simulink model "ACCfinall"  (Simulink 8.4)
settings: Solver=ode45  StartTime=0.0  StopTime=200.0  RelTol=1e-3
undefined symbols (not defined in the file or in its folder): sigbuilder_block
libraries: simulink x1
settings Model: Creator=asim  LastModifiedBy=asim
settings DataIOCC: SignalLoggingSaveFormat=Dataset
settings OptimizationCC: ExpressionDepthLimit=128
settings DebuggingCC: UnderspecifiedInitializationDetection=Simplified  MergeDetectMultiDrivingBlocksExec=error  SolverPrmCheckMsg=none  FcnCallInpInsideContextMsg=EnableAllAsError  StateNameClashWarn=none
settings GRTTargetCC: CombineOutputUpdateFcns=on  GRTInterface=off

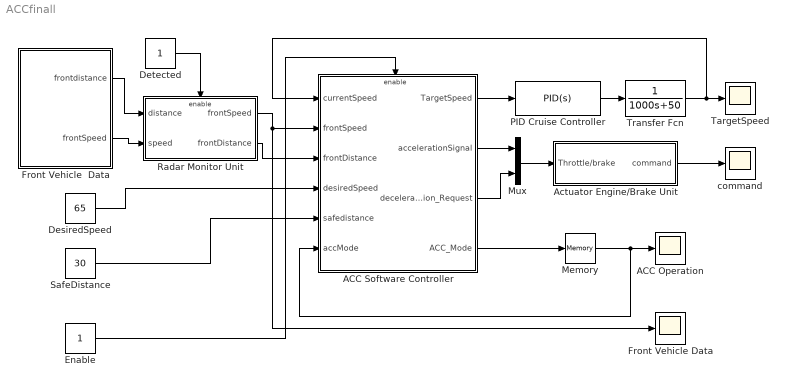
== system ACCfinall ==
  ACC Operation : Scope
      settings: TimeRange=10  YMin=0  YMax=3  SaveName=ScopeData3
  "ACC Software Controller " : Subsystem
  Actuator Engine/Brake Unit : Subsystem
  DesiredSpeed : Constant  Value=65
  "Detected " : Constant
  Enable : Constant
  Front Vehicle  Data : Subsystem  Tag=STV Subsys  LoadFcn=sigbuilder_block('load');  StartFcn=sigbuilder_block('start');  StopFcn=sigbuilder_block('stop');  ClipboardFcn=sigbuilder_block('clipboard');  mask(Sigbuilder block){}
      mask help: Simulink:masks:SigbuilderBlock_MD
      mask init:
      | if ~strcmp(get_param(bdroot(gcbh),'SimulationStatus'),'stopped') tuvar = sigbuilder_block('maskInit'); end
      settings: CopyFcn=sigbuilder_block('copy');  DeleteFcn=sigbuilder_block('delete');  ModelCloseFcn=sigbuilder_block('modelClose');  PreSaveFcn=sigbuilder_block('preSave');  PauseFcn=sigbuilder_block('pause');  ContinueFcn=sigbuilder_block('continue');  NameChangeFcn=sigbuilder_block('namechange');  OpenFcn=sigbuilder_block('open',[410.25 112.5 550.5 394.5 ]);  CloseFcn=sigbuilder_block('close');
      mask Display: plot(0, 0, 100, 100,[2, 2, 32, 32, 2], [68, 8, 8, 68, 68],[32, 2], [38, 38], [32, 19, 2],[53, 60, 44], [32, 17, 17, 2],[16, 16, 31, 31]);txt = getActiveGroup(gcbh);text(2, 100, txt,'verticalAlignment', 'top');
  Front Vehicle Data : Scope
  Memory : Memory  InheritSampleTime=on
  Mux : Mux  Inputs=2
  PID Cruise Controller : simulink/Continuous/PID Controller  Controller=PID  TimeDomain=Continuous-time  SampleTime=-1  IntegratorMethod=Forward Euler  FilterMethod=Forward Euler  Form=Parallel  P=65.9263869879216  I=5.57652865052723  D=-273.538535319166  N=0.241013160763614  InitialConditionSource=internal  InitialConditionForIntegrator=0  InitialConditionForFilter=0  ExternalReset=none  LimitOutput=off  UpperSaturationLimit=inf  LowerSaturationLimit=-inf  LinearizeAsGain=on  AntiWindupMode=none  Kb=1  TrackingMode=off  Kt=1  PParamMin=[]  PParamMax=[]  IParamMin=[]  IParamMax=[]  DParamMin=[]  DParamMax=[]  NParamMin=[]  NParamMax=[]  KbParamMin=[]  KbParamMax=[]  KtParamMin=[]  KtParamMax=[]  POutMin=[]  POutMax=[]  IOutMin=[]  IOutMax=[]  DOutMin=[]  DOutMax=[]  NOutMin=[]  NOutMax=[]  KbOutMin=[]  KbOutMax=[]  KtOutMin=[]  KtOutMax=[]  IntegratorOutMin=[]  IntegratorOutMax=[]  FilterOutMin=[]  FilterOutMax=[]  SumOutMin=[]  SumOutMax=[]  SumI1OutMin=[]  SumI1OutMax=[]  SumI2OutMin=[]  SumI2OutMax=[]  SumI3OutMin=[]  SumI3OutMax=[]  SumDOutMin=[]  SumDOutMax=[]  SaturationOutMin=[]  SaturationOutMax=[]  IntegratorContinuousStateAttributes=''  IntegratorStateMustResolveToSignalObject=off  IntegratorRTWStateStorageClass=Auto  FilterContinuousStateAttributes=''  FilterStateMustResolveToSignalObject=off  FilterRTWStateStorageClass=Auto  DifferentiatorICPrevScaledInput=0  DifferentiatorOutMin=[]  DifferentiatorOutMax=[]  UseFilter=on
  Radar Monitor Unit : Subsystem
  SafeDistance : Constant  Value=30
  TargetSpeed : Scope
      settings: YMin=0  YMax=70
  Transfer Fcn : TransferFcn  Denominator=[1000 50]
  command : Scope
      settings: SaveName=ScopeData2
  wires:
  "ACC Software Controller "/1(TargetSpeed) -> PID Cruise Controller/1
  Transfer Fcn/1 -> TargetSpeed/1, "ACC Software Controller "/1(currentSpeed)
  Radar Monitor Unit/2(frontDistance) -> "ACC Software Controller "/3(frontDistance)
  PID Cruise Controller/1 -> Transfer Fcn/1
  "ACC Software Controller "/4(ACC_Mode) -> Memory/1
  Memory/1 -> ACC Operation/1, "ACC Software Controller "/6(accMode)
  "ACC Software Controller "/2(accelerationSignal) -> Mux/1
  "ACC Software Controller "/3(deceleration_Request) -> Mux/2
  Mux/1 -> Actuator Engine/Brake Unit/1(Throttle/brake)
  Actuator Engine/Brake Unit/1(command) -> command/1
  Front Vehicle  Data/1(frontdistance) -> Radar Monitor Unit/1(distance)
  Radar Monitor Unit/1(frontSpeed) -> "ACC Software Controller "/2(frontSpeed), Front Vehicle Data/1
  DesiredSpeed/1 -> "ACC Software Controller "/4(desiredSpeed)
  SafeDistance/1 -> "ACC Software Controller "/5(safedistance)
  Enable/1 -> "ACC Software Controller "/Enable
  "Detected "/1 -> Radar Monitor Unit/Enable
  Front Vehicle  Data/2(frontSpeed) -> Radar Monitor Unit/2(speed)

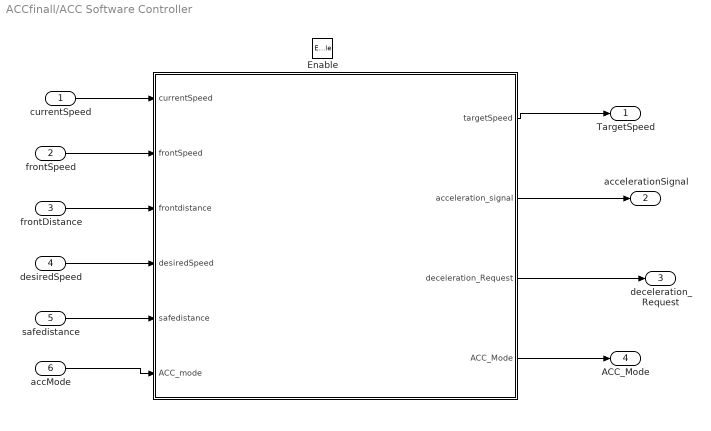
== system ACCfinall/ACC Software Controller  ==
  currentSpeed : Inport
  frontSpeed : Inport  Port=2
  frontDistance : Inport  Port=3
  desiredSpeed : Inport  Port=4
  safedistance : Inport  Port=5
  accMode : Inport  Port=6
  Enable : EnablePort
  "          " : MATLAB Function  TreatAsAtomicUnit=on
  TargetSpeed : Outport
  accelerationSignal : Outport  Port=2
  deceleration_Request : Outport  Port=3
  ACC_Mode : Outport  Port=4
  wires:
  "          "/1(targetSpeed) -> TargetSpeed/1
  currentSpeed/1 -> "          "/1(currentSpeed)
  "          "/2(acceleration_signal) -> accelerationSignal/1
  "          "/4(ACC_Mode) -> ACC_Mode/1
  "          "/3(deceleration_Request) -> deceleration_Request/1
  frontSpeed/1 -> "          "/2(frontSpeed)
  frontDistance/1 -> "          "/3(frontdistance)
  desiredSpeed/1 -> "          "/4(desiredSpeed)
  safedistance/1 -> "          "/5(safedistance)
  accMode/1 -> "          "/6(ACC_mode)

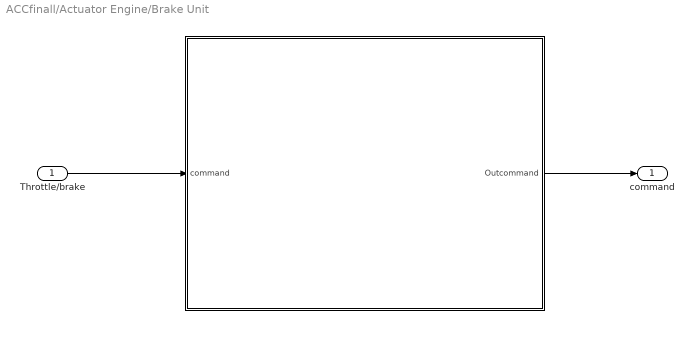
== system ACCfinall/Actuator Engine/Brake Unit ==
  Throttle/brake : Inport
  "          " : MATLAB Function  TreatAsAtomicUnit=on
  command : Outport
  wires:
  "          "/1(Outcommand) -> command/1
  Throttle/brake/1 -> "          "/1(command)

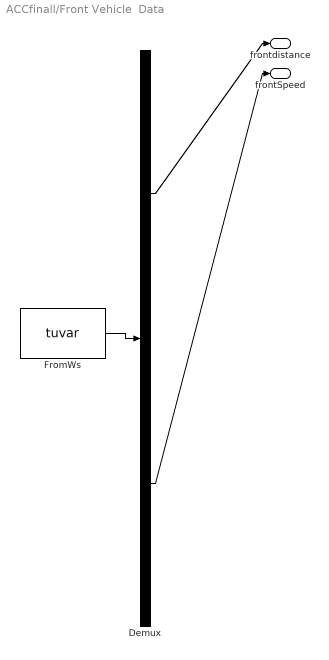
== system ACCfinall/Front Vehicle  Data ==
  Demux : Demux  Tag=STV Demux  Outputs=2
  FromWs : FromWorkspace  Tag=STV FromWs  VariableName=tuvar  SampleTime=0  SigBuilderData=DataTag0  VnvData=DataTag1
      SigBuilderData=|
      | common.afterFinalStr = 'Extrapolate'
      | common.sampleTime = 0
      | dataSet.timeRange = [10 100]
      | dataSet.name = 'Front Vehicle '
      | sbobj.Groups.Name = 'Front Vehicle '
      | sbobj.Groups.Signals(1).Name = 'frontdistance'
      | sbobj.Groups.Signals(1).XData = [10 11 11 12 12 13 13 14 14 15 15 16 16 17 17 18 18 19 19 20 20 21 21 22 22 23 23 24 24 25 25 26 26 27 27 28 28 29 29 30 30 31 31 32 32 33 33 34 34 35 35 36 36 37 37 38 38 39 39 40 40 41 41 42 42 43 43 44 44 45 45 46 46 47 47 48 48 49 49 50 50 51 51 52 52 53 53 54 54 55 55 56 56 57 57 58 58 59 59 60 60 61 61 62 62 63 63 64 64 65 65 66 66 67 67 68 68 69 69 70 70 71 71 72 72 73 73 74 74 75 75 76 76 77 77 78 78 79 79 80 80 81 81 82 82 83 83 84 84 85 85 86 86 87 87 88 88 89 89 90 90 91 91 92 92 93 93 94 94 95 95 96 96 97 97 98 98 99 99 100]
      | sbobj.Groups.Signals(1).YData = [0 40 0 40 0 40 0 40 0 40 0 40 0 40 0 40 0 40 0 40 0 40 0 40 0 40 0 40 0 40 0 40 0 40 0 40 0 40 0 40 0 40 0 40 0 40 0 40 0 40 0 40 0 40 0 40 0 40 0 40 0 40 0 40 0 40 0 40 0 40 0 40 0 40 0 40 0 40 0 40 0 40 0 40 0 40 0 40 0 40 0 40 0 40 0 40 0 40 0 40 0 40 0 40 0 40 0 40 0 40 0 40 0 40 0 40 0 40 0 40 0 40 0 40 0 40 0 40 0 40 0 40 0 40 0 40 0 40 0 40 0 40 0 40 0 40 0 40 0 40 0 40 0 40 0 40 0 40 0 40 0 40 0 40 0 40 0 40 0 40 0 40 0 40 0 40 0 40 0 40]
      | sbobj.Groups.Signals(2).Name = 'frontSpeed'
      | sbobj.Groups.Signals(2).XData = [10 46 46 64 64 100]
      | sbobj.Groups.Signals(2).YData = [20.5 41.4 24.2 51.2 30.2 68]
      | sbobj.Groups.TimeRange = [10 100]
  frontdistance : Outport  Tag=STV Outport
  frontSpeed : Outport  Tag=STV Outport  Port=2
  wires:
  FromWs/1 -> Demux/1
  Demux/1 -> frontdistance/1
  Demux/2 -> frontSpeed/1

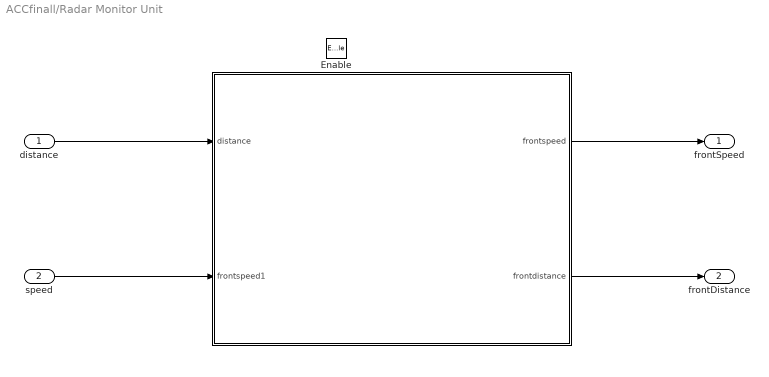
== system ACCfinall/Radar Monitor Unit ==
  distance : Inport
  speed : Inport  Port=2
  Enable : EnablePort
  "          " : MATLAB Function  TreatAsAtomicUnit=on
  frontSpeed : Outport
  frontDistance : Outport  Port=2
  wires:
  "          "/1(frontspeed) -> frontSpeed/1
  distance/1 -> "          "/1(distance)
  speed/1 -> "          "/2(frontspeed1)
  "          "/2(frontdistance) -> frontDistance/1

== matlab function ACC Software Controller /           ==
  data: currentSpeed input double; frontSpeed input double; frontdistance input double; desiredSpeed input double; safedistance input double; targetSpeed output double; acceleration_signal output double; deceleration_Request output double; ACC_Mode output double; ACC_mode input double

% This model is free model: you can redistribute it and/or modify
% it under the terms of the General Public License. 
% This funciton is updated from the project AutoPlug-3.0. 
% Authors: Asim Abdulkhaleq and Stefan Wagner 
% 2015

function [targetSpeed, acceleration_signal, deceleration_Request, ACC_Mode]  = ACC_Software_Controller(currentSpeed, frontSpeed, frontdistance,desiredSpeed, safedistance, ACC_mode)
timeC=0.2;
acc_C = 8.5;
accel_cmd=0;
decel_cmd=0;
 
persistent setSpeed;
if isempty(setSpeed)
    setSpeed= 0;
end
 minSpeed=10;
 
deltaX=((frontSpeed*frontSpeed)-(currentSpeed*currentSpeed))/(2*(-acc_C));


if(frontdistance<=(safedistance + (deltaX)))
    if(frontdistance <= deltaX + safedistance) && (frontdistance  >= safedistance)
        
        tmpSpeed1 = sqrt(abs(currentSpeed * currentSpeed) + abs(2*(-acc_C)*abs((deltaX + safedistance)-frontdistance)));
        setSpeed = max(frontSpeed,tmpSpeed1);      % stops the reduction at front_speed.
        accel_cmd=1;
        decel_cmd=0;
         ACC_mode=1;
    elseif(frontdistance <safedistance)
        tmpSpeed2 = sqrt(abs(currentSpeed * currentSpeed) + abs(2*(-acc_C)*abs(safedistance-frontdistance)));
        setSpeed = max(minSpeed,tmpSpeed2);
       accel_cmd=0;
       decel_cmd=1;
        ACC_mode=2;
    end
elseif(frontdistance>(safedistance + (deltaX)))
    setSpeed = currentSpeed + (acc_C*timeC);% v = u + at
    %setSpeed = min(desiredSpeed,tmpSpeed3);
     accel_cmd=1;
     decel_cmd=0;
     ACC_mode=3;
    
end
 setSpeed = min(desiredSpeed,setSpeed);
 
 targetSpeed = setSpeed - currentSpeed;
ACC_Mode=ACC_mode;
acceleration_signal=accel_cmd;
deceleration_Request=decel_cmd;

end

== matlab function Actuator Engine//Brake Unit/           ==
  data: command input double; Outcommand output double
function Outcommand   = ActuatorsUnit(command)
 
 Outcommand=command;
  
end

== matlab function Radar Monitor Unit/           ==
  data: frontspeed output double; frontdistance output double; distance input double; frontspeed1 input double
function [frontspeed,frontdistance]  = RadarUnit(distance, frontspeed1)
 
 frontspeed=frontspeed1;
 fprintf('m = %f\n', frontspeed); 
 frontdistance=distance;
 fprintf('x = %f\n', frontdistance); 
end
